simulink model "P_Control"  (R2018a)
settings: Solver=VariableStepAuto  StartTime=0.0  StopTime=2  RelTol=1e-3
undefined symbols (not defined in the file): A, b, beta, Kv, L, m, P_r, P_s, V0, wn, zeta
libraries: simulink x1
settings Model: Creator=UFUK  LastModifiedBy=UFUK

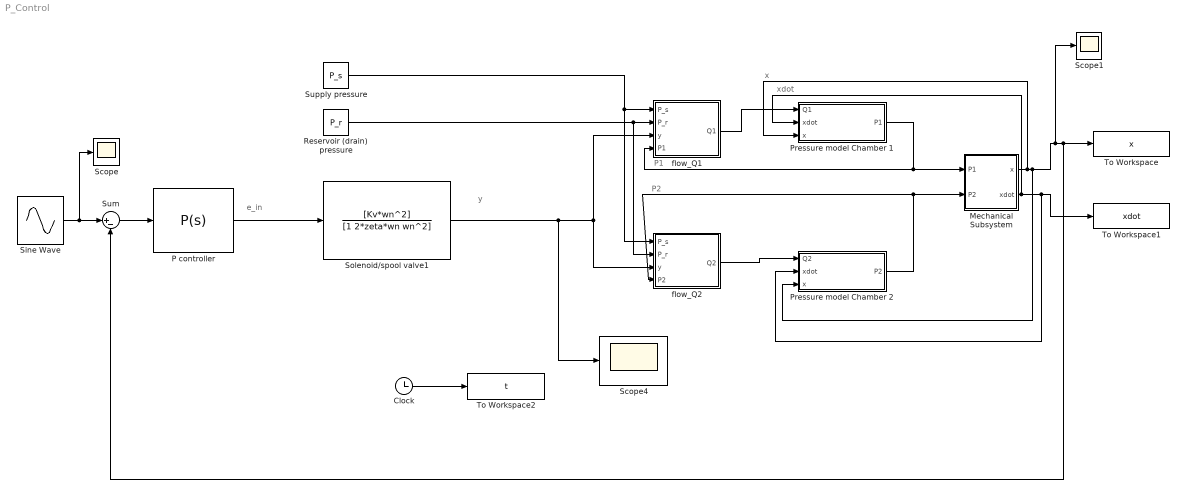
== system P_Control ==
  note: xdot
  note: x
  note: y
  note: P2
  note: P1
  note: e_in
  " flow_Q2" : MATLAB Function  TreatAsAtomicUnit=on
  Clock : Clock
  Mechanical Subsystem : Subsystem
  P controller : simulink/Continuous/PID Controller  Controller=P  TimeDomain=Continuous-time  SampleTime=-1  IntegratorMethod=Forward Euler  FilterMethod=Forward Euler  Form=Parallel  UseFilter=on  ControllerParametersSource=internal  P=352.94  I=1  D=0  N=100  InitialConditionSource=internal  InitialConditionForIntegrator=0  InitialConditionForFilter=0  ExternalReset=none  LimitOutput=off  UpperSaturationLimit=inf  LowerSaturationLimit=-inf  LinearizeAsGain=on  AntiWindupMode=none  Kb=1  TrackingMode=off  Kt=1  PParamMin=[]  PParamMax=[]  IParamMin=[]  IParamMax=[]  DParamMin=[]  DParamMax=[]  NParamMin=[]  NParamMax=[]  KbParamMin=[]  KbParamMax=[]  KtParamMin=[]  KtParamMax=[]  POutMin=[]  POutMax=[]  IOutMin=[]  IOutMax=[]  DOutMin=[]  DOutMax=[]  NOutMin=[]  NOutMax=[]  KbOutMin=[]  KbOutMax=[]  KtOutMin=[]  KtOutMax=[]  IntegratorOutMin=[]  IntegratorOutMax=[]  FilterOutMin=[]  FilterOutMax=[]  SumOutMin=[]  SumOutMax=[]  SumI1OutMin=[]  SumI1OutMax=[]  SumI2OutMin=[]  SumI2OutMax=[]  SumI3OutMin=[]  SumI3OutMax=[]  SumDOutMin=[]  SumDOutMax=[]  SaturationOutMin=[]  SaturationOutMax=[]  IntegratorContinuousStateAttributes=''  IntegratorStateMustResolveToSignalObject=off  IntegratorRTWStateStorageClass=Auto  FilterContinuousStateAttributes=''  FilterStateMustResolveToSignalObject=off  FilterRTWStateStorageClass=Auto  DifferentiatorICPrevScaledInput=0  DifferentiatorOutMin=[]  DifferentiatorOutMax=[]  FilterDiffOutCoefMin=[]  FilterDiffOutCoefMax=[]  SumDenOutMin=[]  SumDenOutMax=[]  SumNumOutMin=[]  SumNumOutMax=[]  ReciprocalOutMin=[]  ReciprocalOutMax=[]  DivideOutMin=[]  DivideOutMax=[]  TunerSelectOption=Transfer Function Based (PID Tuner App)
  Pressure model Chamber 1 : Subsystem
  Pressure model Chamber 2 : Subsystem
  Reservoir (drain) pressure : Constant  Value=P_r
  Scope : Scope
  Scope1 : Scope
  Scope4 : Scope
  Sine Wave : Sin  Amplitude=L/4  Bias=L/2  Frequency=12.57  SampleTime=0
  Solenoid/spool valve1 : TransferFcn  Numerator=[Kv*wn^2]  Denominator=[1 2*zeta*wn wn^2]
  Sum : Sum  Inputs=|+-
  Supply pressure : Constant  Value=P_s
  To Workspace : ToWorkspace  VariableName=x  SaveFormat=Timeseries  SampleTime=-1
  To Workspace1 : ToWorkspace  VariableName=xdot  SaveFormat=Timeseries  SampleTime=-1
  To Workspace2 : ToWorkspace  VariableName=t  SaveFormat=Timeseries  SampleTime=-1
  flow_Q1 : MATLAB Function  TreatAsAtomicUnit=on
  wires:
  Mechanical Subsystem/2(xdot) -> To Workspace1/1, Pressure model Chamber 2/2(xdot), Pressure model Chamber 1/2(xdot)
  P controller/1 -> Solenoid/spool valve1/1
  Reservoir (drain) pressure/1 -> " flow_Q2"/2(P_r), flow_Q1/2(P_r)
  Sum/1 -> P controller/1
  Sine Wave/1 -> Scope/1, Sum/1
  " flow_Q2"/1(Q2) -> Pressure model Chamber 2/1(Q2)
  Mechanical Subsystem/1(x) -> Scope1/1, Sum/2, To Workspace/1, Pressure model Chamber 2/3(x), Pressure model Chamber 1/3(x)
  Supply pressure/1 -> " flow_Q2"/1(P_s), flow_Q1/1(P_s)
  Pressure model Chamber 1/1(P1) -> flow_Q1/4(P1), Mechanical Subsystem/1(P1)
  flow_Q1/1(Q1) -> Pressure model Chamber 1/1(Q1)
  Pressure model Chamber 2/1(P2) -> Mechanical Subsystem/2(P2), " flow_Q2"/4(P2)
  Clock/1 -> To Workspace2/1
  Solenoid/spool valve1/1 -> Scope4/1, flow_Q1/3(y), " flow_Q2"/3(y)

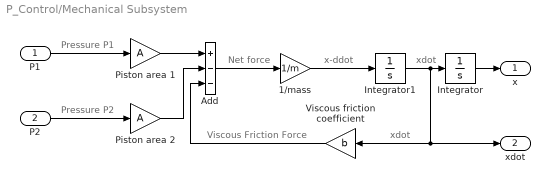
== system P_Control/Mechanical Subsystem ==
  note: xdot
  note: xdot
  note: x-ddot
  note: Net force
  note: Viscous Friction Force
  note: Pressure P2
  note: Pressure P1
  P1 : Inport
  P2 : Inport  Port=2
  1/mass : Gain  Gain=1/m
  Add : Sum  Inputs=+--
  Integrator : Integrator  InitialCondition=L/2
  Integrator1 : Integrator
  Piston area 1 : Gain  Gain=A
  Piston area 2 : Gain  Gain=A
  Viscous friction coefficient : Gain  Gain=b
  x : Outport  VectorParamsAs1DForOutWhenUnconnected=on
  xdot : Outport  Port=2  VectorParamsAs1DForOutWhenUnconnected=on
  wires:
  P2/1 -> Piston area 2/1
  P1/1 -> Piston area 1/1
  Piston area 1/1 -> Add/1
  Piston area 2/1 -> Add/2
  Add/1 -> 1/mass/1
  1/mass/1 -> Integrator1/1
  Integrator1/1 -> Integrator/1, xdot/1, Viscous friction coefficient/1
  Integrator/1 -> x/1
  Viscous friction coefficient/1 -> Add/3

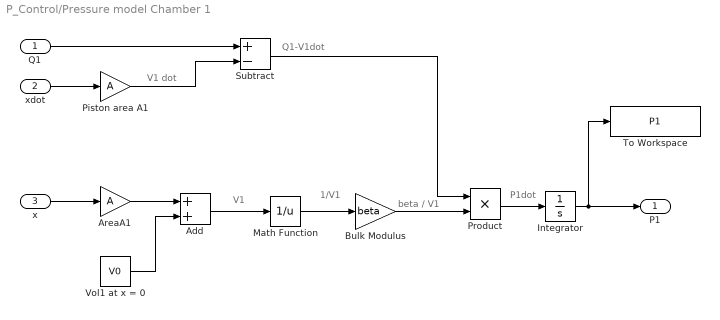
== system P_Control/Pressure model Chamber 1 ==
  note: P1dot
  note: beta / V1
  note: 1/V1
  note: V1
  note: Q1-V1dot
  note: V1 dot
  Q1 : Inport
  xdot : Inport  Port=2
  x : Inport  Port=3
  Add : Sum
  AreaA1 : Gain  Gain=A
  Bulk Modulus : Gain  Gain=beta
  Integrator : Integrator  InitialCondition=0.1*P_s
  Math Function : Math  Operator=reciprocal  SaturateOnIntegerOverflow=on
  Piston area A1 : Gain  Gain=A
  Product : Product
  Subtract : Sum  Inputs=+-
  To Workspace : ToWorkspace  VariableName=P1  SaveFormat=Timeseries  SampleTime=-1
  Vol1 at x = 0 : Constant  Value=V0
  P1 : Outport  VectorParamsAs1DForOutWhenUnconnected=on
  wires:
  Q1/1 -> Subtract/1
  xdot/1 -> Piston area A1/1
  Piston area A1/1 -> Subtract/2
  x/1 -> AreaA1/1
  AreaA1/1 -> Add/1
  Subtract/1 -> Product/1
  Math Function/1 -> Bulk Modulus/1
  Add/1 -> Math Function/1
  Product/1 -> Integrator/1
  Integrator/1 -> To Workspace/1, P1/1
  Vol1 at x = 0/1 -> Add/2
  Bulk Modulus/1 -> Product/2

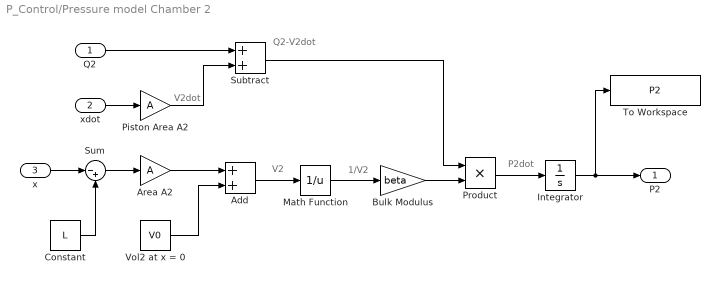
== system P_Control/Pressure model Chamber 2 ==
  note: P2dot
  note: 1/V2
  note: V2
  note: Q2-V2dot
  note: V2dot
  Q2 : Inport
  xdot : Inport  Port=2
  x : Inport  Port=3
  Add : Sum
  Area A2 : Gain  Gain=A
  Bulk Modulus : Gain  Gain=beta
  Constant : Constant  Value=L
  Integrator : Integrator  InitialCondition=0.1*P_s
  Math Function : Math  Operator=reciprocal  SaturateOnIntegerOverflow=on
  Piston Area A2 : Gain  Gain=A
  Product : Product
  Subtract : Sum
  Sum : Sum  Inputs=|-+
  To Workspace : ToWorkspace  VariableName=P2  SaveFormat=Timeseries  SampleTime=-1
  Vol2 at x = 0 : Constant  Value=V0
  P2 : Outport  VectorParamsAs1DForOutWhenUnconnected=on
  wires:
  xdot/1 -> Piston Area A2/1
  Add/1 -> Math Function/1
  Math Function/1 -> Bulk Modulus/1
  Bulk Modulus/1 -> Product/2
  Area A2/1 -> Add/1
  Q2/1 -> Subtract/1
  Piston Area A2/1 -> Subtract/2
  Subtract/1 -> Product/1
  Product/1 -> Integrator/1
  Integrator/1 -> To Workspace/1, P2/1
  Vol2 at x = 0/1 -> Add/2
  Sum/1 -> Area A2/1
  Constant/1 -> Sum/2
  x/1 -> Sum/1

== matlab function P_Control/ flow_Q2 ==
  data: P_s input; Q2 output; P_r input; y input; P2 input
% flow_Q2.m
%
% This M-file models the volumetric-flow rate of fluid in/out of chamber 2.
% Assumes valve flow is modeled by flow through a sharp-edged orifice
%
% Inputs: u (4x1 vector) = [ P_s P_r y P2 ]'
% P_s = supply pressure, Pa
% P_r = reservoir pressure (drain), Pa
% y = valve displacement, m
% P2 = pressure of chamber 2, Pa
%
% Output: Q2= in/out volumetric-flow rate, m^3/s
%

function Q2 = flow_Q2(P_s, P_r, y, P2)
u = [P_s P_r y P2]';
%system parameter
h = 0.0092; %height of the valve opening,m

%hydraulic constants
Cd = 0.62; %discharge coefficient
rho = 896; %fluid density, kg/m^3

%System inputs
P_s = u(1); % supply pressure, Pa
P_r = u(2); %reservoir pressure, Pa
y = u(3); %valve displacement, m
P1 = u(4); % pressure in chamber 1, Pa

%Compute valve orifice area
Av = abs(y)*h; %valve orifice area, m^2

% Determine if flow is from supply (y > 0), or if flow
% is out to reservoir pressure (y < 0)
if y <= 0
    % Chamber 2 is connected to the supply, P_s
    % (flow is positive if P_s > P1)
    Q2 = Cd*Av*sign(P_s - P2)*sqrt(2*abs(P_s - P2)/rho);
else
    % Chamber 2 is connected to the reservoir, P_r
    % (flow is negative if P2 > P_r)
    Q2 = -Cd*Av*sign(P2 - P_r)*sqrt(2*abs(P2 - P_r)/rho);
end
y=u;

== matlab function P_Control/flow_Q1 ==
  data: P_s input; Q1 output; P_r input; y input; P1 input
% flow_Q1.m
%
% This M-file models the volumetric-flow rate of fluid in/out of chamber 1.
% Assumes valve flow is modeled by flow through a sharp-edged orifice
%
% Inputs: u (4x1 vector) = [ P_s P_r y P1 ]'
% P_s = supply pressure, Pa
% P_r = reservoir pressure (drain), Pa
% y = valve displacement, m
% P1 = pressure of chamber 1, Pa
%
% Output: Q1 = in/out volumetric-flow rate, m^3/s
%
function Q1 = flow_Q1(P_s,P_r,y,P1)
u = [P_s P_r y P1]';
%system parameter
h = 0.0092; %height of the valve opening,m

%hydraulic constants
Cd = 0.62; %discharge coefficient
rho = 896; %fluid density, kg/m^3

%System inputs
P_s = u(1); % supply pressure, Pa
P_r = u(2); %reservoir pressure, Pa
y = u(3); %valve displacement, m
P1 = u(4); % pressure in chamber 1, Pa

%Compute valve orifice area
Av = abs (y)*h; %valve orifice area, m^2

% Determine if flow is from supply (y > 0), or if flow
% is out to reservoir pressure (y < 0)
if y >= 0
    % Chamber 1 is connected to the supply, P_s
    % (flow is positive if P_s > P1)
    Q1 = Cd*Av*sign(P_s - P1)*sqrt(2*abs(P_s - P1)/rho);
else
    % Chamber 1 is connected to the reservoir, P_r
    % (flow is negative if P1 > P_r)
    Q1 = -Cd*Av*sign(P1 - P_r)*sqrt(2*abs(P1 - P_r)/rho);
end
y = u;
